simulink subsystem "TrajandControl"  (R2022a)
settings: Solver=VariableStepAuto  StartTime=0.0  StopTime=10.0  RelTol=1e-3
values from neighbouring files (symbols this model uses):
  kd_altitude = 0.475    [QuadcopterParameters.m]    (also in QuadcopterParameters1.m)
  kd_attitude = 20    [QuadcopterParameters.m]    (also in QuadcopterParameters1.m)
  KD_position = 0.85    [QuadcopterParameters.m]    (also in QuadcopterParameters1.m)
  ki_altitude = 0.275    [QuadcopterParameters.m]    (also in QuadcopterParameters1.m)
  ki_attitude = 0.01    [QuadcopterParameters.m]    (also in QuadcopterParameters1.m)
  KP_altitude = 0.8    [QuadcopterParameters.m]    (also in QuadcopterParameters1.m)
  kp_attitude = 1    [QuadcopterParameters.m]    (also in QuadcopterParameters1.m)
  KP_position = 0.1    [QuadcopterParameters.m]    (also in QuadcopterParameters1.m)
libraries: nesl_utility x6, slpidlib x4, sm_lib x1
settings Model: Creator=ADMIN  LastModifiedBy=ADMIN

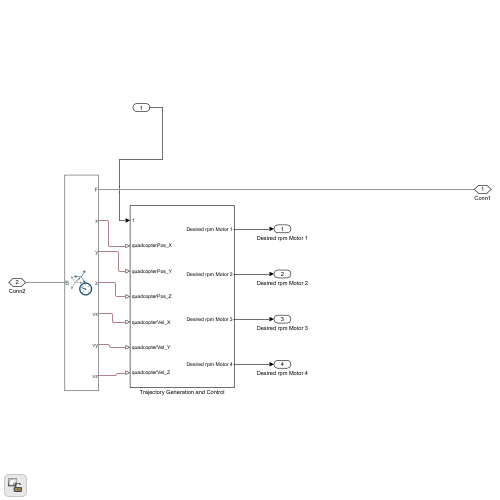
[thumbnail: Simulink's stored preview of the top-level diagram]
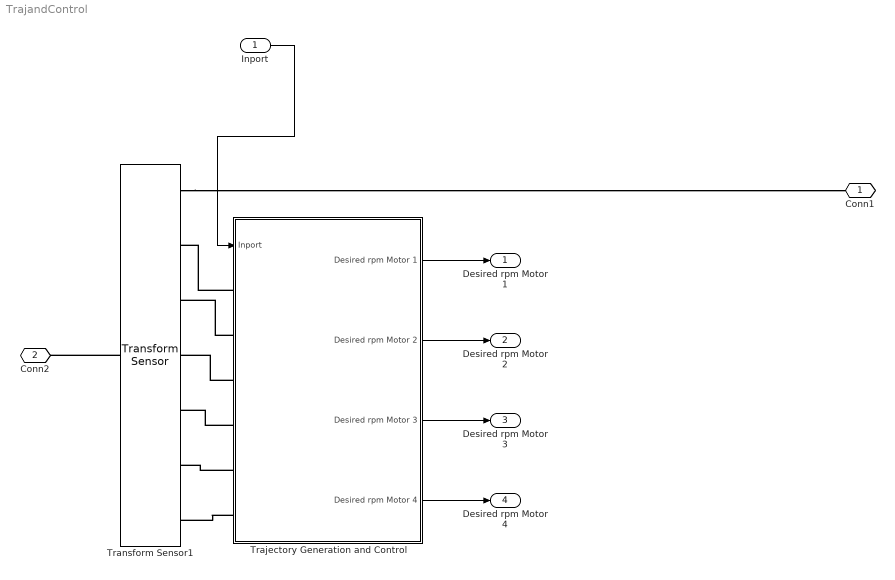
== system TrajandControl ==
  Inport : Inport
  Trajectory Generation and Control : Subsystem
  Transform Sensor1 : sm_lib/Frames and Transforms/Transform Sensor  MeasurementFrame=NonRotatingBase  SenseAngle=off  SenseAxis=off  SenseAngle1=off  SenseAngle2=off  SenseAngle3=off  SenseQ=off  SenseR=off  SenseOmegaX=off  SenseOmegaY=off  SenseOmegaZ=off  SenseOmega1=off  SenseOmega2=off  SenseOmega3=off  SenseQDot=off  SenseRDot=off  SenseAlphaX=off  SenseAlphaY=off  SenseAlphaZ=off  SenseAlpha1=off  SenseAlpha2=off  SenseAlpha3=off  SenseQDDot=off  SenseRDDot=off  SenseX=on  SenseY=on  SenseZ=on  SenseRad=off  SenseAzim=off  SenseDist=off  SenseInc=off  SenseXDot=on  SenseYDot=on  SenseZDot=on  SenseRadDot=off  SenseAzimDot=off  SenseDistDot=off  SenseIncDot=off  SenseXDDot=off  SenseYDDot=off  SenseZDDot=off  SenseRadDDot=off  SenseAzimDDot=off  SenseDistDDot=off  SenseIncDDot=off
  Conn1 : PMIOPort  Side=Right
  Conn2 : PMIOPort  Port=2  Side=Left
  Desired rpm Motor 1 : Outport
  Desired rpm Motor 2 : Outport  Port=2
  Desired rpm Motor 3 : Outport  Port=3
  Desired rpm Motor 4 : Outport  Port=4
  wires:
  Trajectory Generation and Control/2(Desired rpm Motor 2) -> Desired rpm Motor 2/1
  Inport/1 -> Trajectory Generation and Control/1(Inport)
  Trajectory Generation and Control/1(Desired rpm Motor 1) -> Desired rpm Motor 1/1
  Trajectory Generation and Control/3(Desired rpm Motor 3) -> Desired rpm Motor 3/1
  Trajectory Generation and Control/4(Desired rpm Motor 4) -> Desired rpm Motor 4/1
  connections:
  Trajectory Generation and Control/LConn1 -- Transform Sensor1/RConn2
  Trajectory Generation and Control/LConn5 -- Transform Sensor1/RConn6
  Trajectory Generation and Control/LConn3 -- Transform Sensor1/RConn4
  Trajectory Generation and Control/LConn2 -- Transform Sensor1/RConn3
  Trajectory Generation and Control/LConn6 -- Transform Sensor1/RConn7
  Trajectory Generation and Control/LConn4 -- Transform Sensor1/RConn5
  Transform Sensor1/LConn1 -- Conn2/RConn1
  Transform Sensor1/RConn1 -- Conn1/RConn1

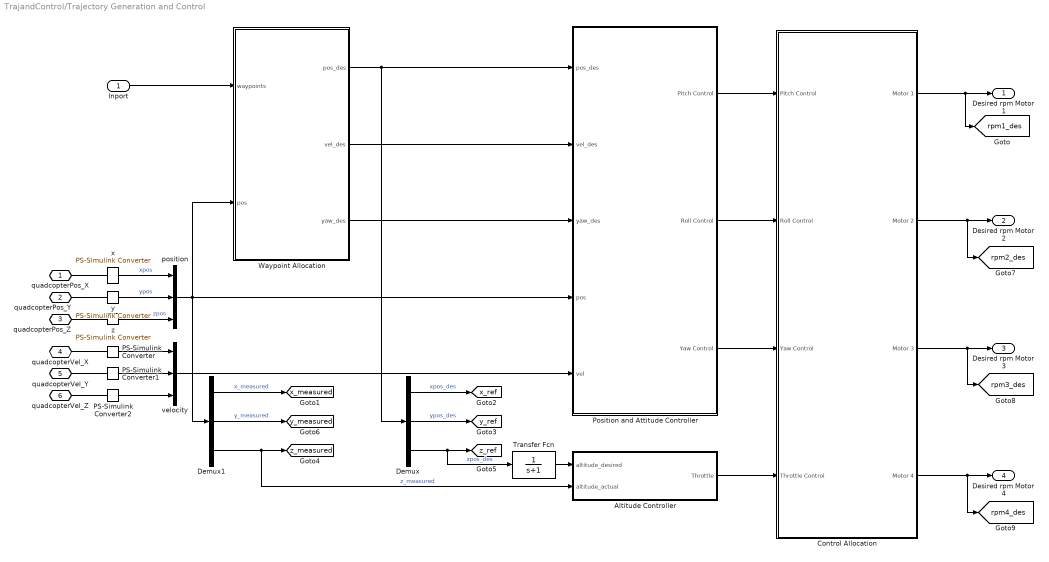
== system TrajandControl/Trajectory Generation and Control ==
  Inport : Inport
  Altitude Controller : Subsystem
  Control Allocation : Subsystem
  Demux : Demux  Outputs=3
  Demux1 : Demux  Outputs=3
  PS-Simulink Converter : nesl_utility/PS-Simulink Converter  PhysicalDomain=network_engine_domain  SubClassName=ps_output  LeftPortType=input  RightPortType=output  PseudoPeriodic=off  Frequencies=[]  VectorFormat=1-D array  Unit=inherit  AffineConversion=off
      settings: SourceProductBaseCode=SS,PW,VE
  PS-Simulink Converter1 : nesl_utility/PS-Simulink Converter  PhysicalDomain=network_engine_domain  SubClassName=ps_output  LeftPortType=input  RightPortType=output  PseudoPeriodic=off  Frequencies=[]  VectorFormat=1-D array  Unit=inherit  AffineConversion=off
      settings: SourceProductBaseCode=SS,PW,VE
  PS-Simulink Converter2 : nesl_utility/PS-Simulink Converter  PhysicalDomain=network_engine_domain  SubClassName=ps_output  LeftPortType=input  RightPortType=output  PseudoPeriodic=off  Frequencies=[]  VectorFormat=1-D array  Unit=inherit  AffineConversion=off
      settings: SourceProductBaseCode=SS,PW,VE
  Position and Attitude Controller : Subsystem
  Transfer Fcn : TransferFcn  Denominator=[1 1]
  Waypoint Allocation : MATLAB Function  TreatAsAtomicUnit=on
  position : Mux  Inputs=3
  velocity : Mux  Inputs=3
  x : nesl_utility/PS-Simulink Converter  PhysicalDomain=network_engine_domain  SubClassName=ps_output  LeftPortType=input  RightPortType=output  PseudoPeriodic=off  Frequencies=[]  VectorFormat=1-D array  Unit=1  AffineConversion=off
      settings: SourceProductBaseCode=SS,PW,VE
  y : nesl_utility/PS-Simulink Converter  PhysicalDomain=network_engine_domain  SubClassName=ps_output  LeftPortType=input  RightPortType=output  PseudoPeriodic=off  Frequencies=[]  VectorFormat=1-D array  Unit=1  AffineConversion=off
      settings: SourceProductBaseCode=SS,PW,VE
  z : nesl_utility/PS-Simulink Converter  PhysicalDomain=network_engine_domain  SubClassName=ps_output  LeftPortType=input  RightPortType=output  PseudoPeriodic=off  Frequencies=[]  VectorFormat=1-D array  Unit=1  AffineConversion=off
      settings: SourceProductBaseCode=SS,PW,VE
  quadcopterPos_X : PMIOPort  Side=Left
  quadcopterPos_Y : PMIOPort  Port=2  Side=Left
  quadcopterPos_Z : PMIOPort  Port=3  Side=Left
  quadcopterVel_X : PMIOPort  Port=4  Side=Left
  quadcopterVel_Y : PMIOPort  Port=5  Side=Left
  quadcopterVel_Z : PMIOPort  Port=6  Side=Left
  Desired rpm Motor 1 : Outport
  Desired rpm Motor 2 : Outport  Port=2
  Desired rpm Motor 3 : Outport  Port=3
  Desired rpm Motor 4 : Outport  Port=4
  tag scope: rpm1_des=global, rpm2_des=global, rpm3_des=global, rpm4_des=global, x_measured=global, x_ref=global, y_measured=global, y_ref=global, z_measured=global, z_ref=global
  wires:
  Control Allocation/4(Motor 4) -> Desired rpm Motor 4/1, [rpm4_des]
  Control Allocation/3(Motor 3) -> Desired rpm Motor 3/1, [rpm3_des]
  Control Allocation/1(Motor 1) -> [rpm1_des], Desired rpm Motor 1/1
  Transfer Fcn/1 -> Altitude Controller/1(altitude_desired)
  Inport/1 -> Waypoint Allocation/1(waypoints)
  Altitude Controller/1(Throttle) -> Control Allocation/4(Throttle Control)
  Position and Attitude Controller/3(Yaw Control) -> Control Allocation/3(Yaw Control)
  Position and Attitude Controller/1(Pitch Control) -> Control Allocation/1(Pitch Control)
  Position and Attitude Controller/2(Roll Control) -> Control Allocation/2(Roll Control)
  Waypoint Allocation/1(pos_des) -> Demux/1, Position and Attitude Controller/1(pos_des)
  Waypoint Allocation/2(vel_des) -> Position and Attitude Controller/2(vel_des)
  Waypoint Allocation/3(yaw_des) -> Position and Attitude Controller/3(yaw_des)
  Control Allocation/2(Motor 2) -> Desired rpm Motor 2/1, [rpm2_des]
  velocity/1 -> Position and Attitude Controller/5(vel)
  Demux1/2 -> [y_measured]  "y_measured"
  Demux1/3 -> Altitude Controller/2(altitude_actual), [z_measured]  "z_measured"
  Demux1/1 -> [x_measured]  "x_measured"
  y/1 -> position/2  "ypos"
  Demux/3 -> [z_ref], Transfer Fcn/1  "zpos_des"
  Demux/1 -> [x_ref]  "xpos_des"
  Demux/2 -> [y_ref]  "ypos_des"
  position/1 -> Position and Attitude Controller/4(pos), Demux1/1, Waypoint Allocation/2(pos)
  x/1 -> position/1  "xpos"
  PS-Simulink Converter2/1 -> velocity/3
  PS-Simulink Converter/1 -> velocity/1
  PS-Simulink Converter1/1 -> velocity/2
  z/1 -> position/3  "zpos"
  connections:
  quadcopterVel_Z/RConn1 -- PS-Simulink Converter2/LConn1
  PS-Simulink Converter1/LConn1 -- quadcopterVel_Y/RConn1
  z/LConn1 -- quadcopterPos_Z/RConn1
  PS-Simulink Converter/LConn1 -- quadcopterVel_X/RConn1
  x/LConn1 -- quadcopterPos_X/RConn1
  y/LConn1 -- quadcopterPos_Y/RConn1

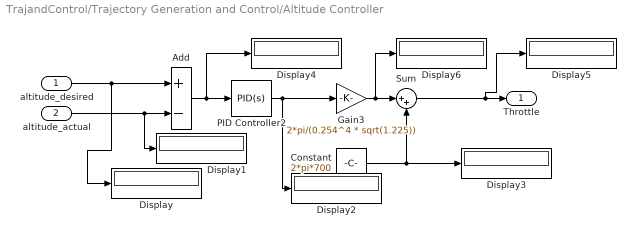
== system TrajandControl/Trajectory Generation and Control/Altitude Controller ==
  altitude_desired : Inport
  altitude_actual : Inport  Port=2
  Add : Sum  Inputs=+-
  Constant : Constant  Value=2*pi*700
  Display{,1..6} (7 alike) : Display
  Gain3 : Gain  Gain=2*pi/(0.254^4 * sqrt(1.225))
  PID Controller2 : slpidlib/PID Controller  Controller=PID  Form=Parallel  TimeDomain=Continuous-time  UseExternalTs=off  SampleTime=-1  IntegratorMethod=Forward Euler  FilterMethod=Forward Euler  ControllerParametersSource=internal  P=KP_altitude  I=ki_altitude  UseKiTs=off  D=kd_altitude  N=1000  UseFilter=on  TunerSelectOption=Transfer Function Based (PID Tuner App)  InitialConditionSource=internal  InitialConditionForIntegrator=0  InitialConditionForFilter=0  DifferentiatorICPrevScaledInput=0  ExternalReset=none  TrackingMode=off  Kt=1  LimitOutput=on  SatLimitsSource=internal  UpperSaturationLimit=50  LowerSaturationLimit=0  LinearizeAsGain=on  AntiWindupMode=none  Kb=1  POutMin=[]  POutMax=[]  IOutMin=[]  IOutMax=[]  DOutMin=[]  DOutMax=[]  NOutMin=[]  NOutMax=[]  SumOutMin=[]  SumOutMax=[]  SaturationOutMin=[]  SaturationOutMax=[]  PParamMin=[]  PParamMax=[]  IParamMin=[]  IParamMax=[]  DParamMin=[]  DParamMax=[]  NParamMin=[]  NParamMax=[]  KbParamMin=[]  KbParamMax=[]  KtParamMin=[]  KtParamMax=[]  KbOutMin=[]  KbOutMax=[]  KtOutMin=[]  KtOutMax=[]  IntegratorOutMin=[]  IntegratorOutMax=[]  FilterOutMin=[]  FilterOutMax=[]  SumI1OutMin=[]  SumI1OutMax=[]  SumI2OutMin=[]  SumI2OutMax=[]  SumI3OutMin=[]  SumI3OutMax=[]  SumI4OutMin=[]  SumI4OutMax=[]  SumDOutMin=[]  SumDOutMax=[]  DifferentiatorOutMin=[]  DifferentiatorOutMax=[]  FilterDiffOutCoefMin=[]  FilterDiffOutCoefMax=[]  ReciprocalOutMin=[]  ReciprocalOutMax=[]  SumDenOutMin=[]  SumDenOutMax=[]  SumNumOutMin=[]  SumNumOutMax=[]  DivideOutMin=[]  DivideOutMax=[]  UdiffTsProdOutMin=[]  UdiffTsProdOutMax=[]  NTsProdOutMin=[]  NTsProdOutMax=[]  UintegralTsProdOutMin=[]  UintegralTsProdOutMax=[]  UngainTsProdOutMin=[]  UngainTsProdOutMax=[]  IntegratorContinuousStateAttributes=''  IntegratorStateMustResolveToSignalObject=off  IntegratorRTWStateStorageClass=Auto  FilterContinuousStateAttributes=''  FilterStateMustResolveToSignalObject=off  FilterRTWStateStorageClass=Auto  ParallelPVariant=InternalParameters  IdealPVariant=Disabled  IVariant=InternalParameters  DVariant=InternalParameters  IntegratorVariant=Continuous  SatVariant=Enabled  AWVariant=Passthrough  PCopyVariant=Disabled  TRVariant=Disabled  FdbkBlocksVariant=Forward  IdealPFdbkVariant=Disabled  SatFdbkVariant=Disabled  DerivativeFilterVariant=ContFilter  NVariant=InternalParameters  NCopyVariant=Disabled  FilterICVariant=InternalICsFilter  IntegratorICVariant=InternalICs  ExternalResetVariant=Disabled  TRSumVariant=Passthrough  SumFdbkVariant=Disabled  SumVariant=Sum_PID  TsampFilterVariant=InternalTs  TsampNgainVariant=Passthrough  TsampIntegralVariant=Passthrough  ExternalSaturationOutDataTypeStr=Inherit: Same as second input  aMode=0
  Sum : Sum  Inputs=|++
  Throttle : Outport
  wires:
  Gain3/1 -> Sum/1, Display6/1
  altitude_desired/1 -> Add/1, Display/1
  Add/1 -> PID Controller2/1, Display4/1
  altitude_actual/1 -> Add/2, Display1/1
  PID Controller2/1 -> Gain3/1, Display2/1
  Constant/1 -> Sum/2, Display3/1
  Sum/1 -> Throttle/1, Display5/1

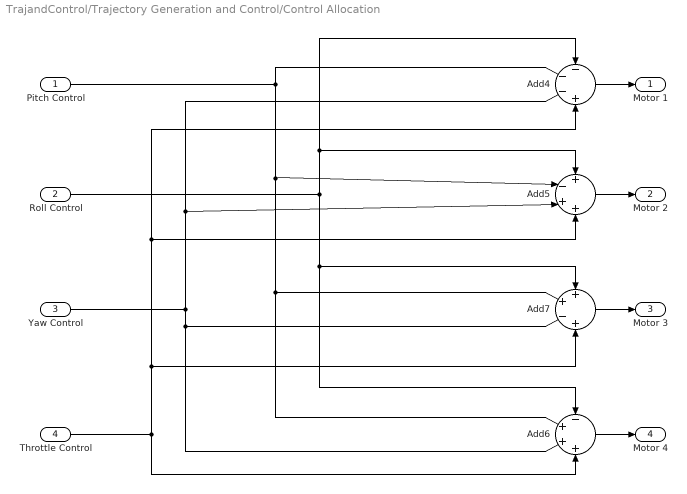
== system TrajandControl/Trajectory Generation and Control/Control Allocation ==
  Pitch Control : Inport
  Roll Control : Inport  Port=2
  Yaw Control : Inport  Port=3
  Throttle Control : Inport  Port=4
  Add4 : Sum  Inputs=---+
  Add5 : Sum  Inputs=+-++
  Add6 : Sum  Inputs=-+++
  Add7 : Sum  Inputs=++-+
  Motor 1 : Outport
  Motor 2 : Outport  Port=2
  Motor 3 : Outport  Port=3
  Motor 4 : Outport  Port=4
  wires:
  Throttle Control/1 -> Add5/4, Add4/4, Add7/4, Add6/4
  Yaw Control/1 -> Add5/3, Add4/3, Add7/3, Add6/3
  Pitch Control/1 -> Add5/2, Add7/2, Add6/2, Add4/2
  Roll Control/1 -> Add7/1, Add6/1, Add5/1, Add4/1
  Add5/1 -> Motor 2/1
  Add4/1 -> Motor 1/1
  Add6/1 -> Motor 4/1
  Add7/1 -> Motor 3/1

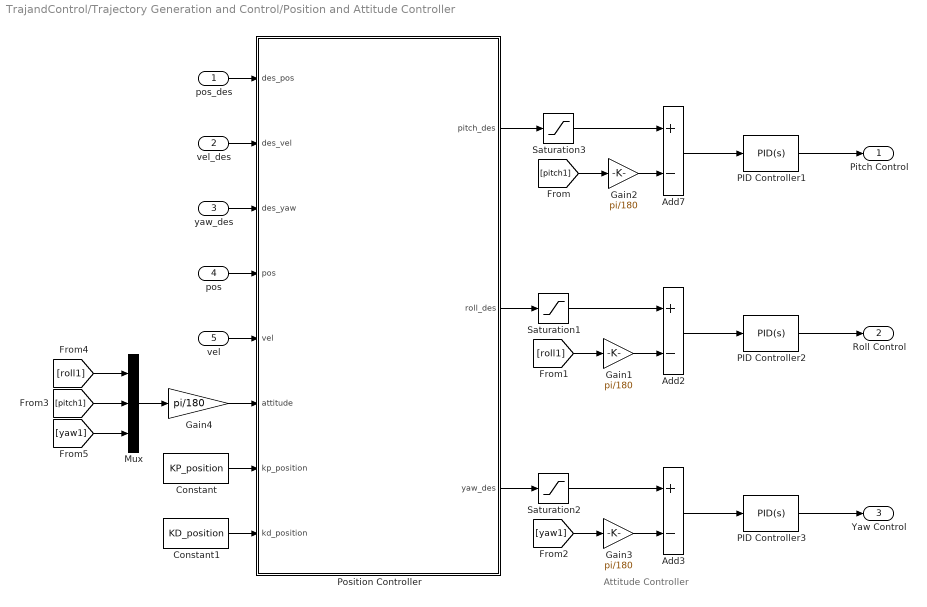
== system TrajandControl/Trajectory Generation and Control/Position and Attitude Controller ==
  note: Attitude Controller
  pos_des : Inport
  vel_des : Inport  Port=2
  yaw_des : Inport  Port=3
  pos : Inport  Port=4
  vel : Inport  Port=5
  Add2 : Sum  Inputs=+-
  Add3 : Sum  Inputs=+-
  Add7 : Sum  Inputs=+-
  Constant : Constant  Value=KP_position
  Constant1 : Constant  Value=KD_position
  Gain{1..4} (4 alike) : Gain  Gain=pi/180
  Mux : Mux  Inputs=3
  PID Controller1 : slpidlib/PID Controller  Controller=PID  Form=Parallel  TimeDomain=Continuous-time  UseExternalTs=off  SampleTime=-1  IntegratorMethod=Forward Euler  FilterMethod=Forward Euler  ControllerParametersSource=internal  P=kp_attitude  I=ki_attitude  UseKiTs=off  D=kd_attitude  N=100  UseFilter=on  TunerSelectOption=Transfer Function Based (PID Tuner App)  InitialConditionSource=internal  InitialConditionForIntegrator=0  InitialConditionForFilter=0  DifferentiatorICPrevScaledInput=0  ExternalReset=none  TrackingMode=off  Kt=1  LimitOutput=on  SatLimitsSource=internal  UpperSaturationLimit=20  LowerSaturationLimit=-20  LinearizeAsGain=on  AntiWindupMode=clamping  Kb=1  POutMin=[]  POutMax=[]  IOutMin=[]  IOutMax=[]  DOutMin=[]  DOutMax=[]  NOutMin=[]  NOutMax=[]  SumOutMin=[]  SumOutMax=[]  SaturationOutMin=[]  SaturationOutMax=[]  PParamMin=[]  PParamMax=[]  IParamMin=[]  IParamMax=[]  DParamMin=[]  DParamMax=[]  NParamMin=[]  NParamMax=[]  KbParamMin=[]  KbParamMax=[]  KtParamMin=[]  KtParamMax=[]  KbOutMin=[]  KbOutMax=[]  KtOutMin=[]  KtOutMax=[]  IntegratorOutMin=[]  IntegratorOutMax=[]  FilterOutMin=[]  FilterOutMax=[]  SumI1OutMin=[]  SumI1OutMax=[]  SumI2OutMin=[]  SumI2OutMax=[]  SumI3OutMin=[]  SumI3OutMax=[]  SumI4OutMin=[]  SumI4OutMax=[]  SumDOutMin=[]  SumDOutMax=[]  DifferentiatorOutMin=[]  DifferentiatorOutMax=[]  FilterDiffOutCoefMin=[]  FilterDiffOutCoefMax=[]  ReciprocalOutMin=[]  ReciprocalOutMax=[]  SumDenOutMin=[]  SumDenOutMax=[]  SumNumOutMin=[]  SumNumOutMax=[]  DivideOutMin=[]  DivideOutMax=[]  UdiffTsProdOutMin=[]  UdiffTsProdOutMax=[]  NTsProdOutMin=[]  NTsProdOutMax=[]  UintegralTsProdOutMin=[]  UintegralTsProdOutMax=[]  UngainTsProdOutMin=[]  UngainTsProdOutMax=[]  IntegratorContinuousStateAttributes=''  IntegratorStateMustResolveToSignalObject=off  IntegratorRTWStateStorageClass=Auto  FilterContinuousStateAttributes=''  FilterStateMustResolveToSignalObject=off  FilterRTWStateStorageClass=Auto  ParallelPVariant=InternalParameters  IdealPVariant=Disabled  IVariant=InternalParameters  DVariant=InternalParameters  IntegratorVariant=Continuous  SatVariant=Enabled  AWVariant=ContClampingParallel  PCopyVariant=Disabled  TRVariant=Disabled  FdbkBlocksVariant=Forward  IdealPFdbkVariant=Disabled  SatFdbkVariant=Disabled  DerivativeFilterVariant=ContFilter  NVariant=InternalParameters  NCopyVariant=Disabled  FilterICVariant=InternalICsFilter  IntegratorICVariant=InternalICs  ExternalResetVariant=Disabled  TRSumVariant=Passthrough  SumFdbkVariant=Disabled  SumVariant=Sum_PID  TsampFilterVariant=InternalTs  TsampNgainVariant=Passthrough  TsampIntegralVariant=Passthrough  ExternalSaturationOutDataTypeStr=Inherit: Same as second input  aMode=0
  PID Controller2 : slpidlib/PID Controller  Controller=PID  Form=Parallel  TimeDomain=Continuous-time  UseExternalTs=off  SampleTime=-1  IntegratorMethod=Forward Euler  FilterMethod=Forward Euler  ControllerParametersSource=internal  P=kp_attitude  I=ki_attitude  UseKiTs=off  D=kd_attitude  N=100  UseFilter=on  TunerSelectOption=Transfer Function Based (PID Tuner App)  InitialConditionSource=internal  InitialConditionForIntegrator=0  InitialConditionForFilter=0  DifferentiatorICPrevScaledInput=0  ExternalReset=none  TrackingMode=off  Kt=1  LimitOutput=on  SatLimitsSource=internal  UpperSaturationLimit=20  LowerSaturationLimit=-20  LinearizeAsGain=on  AntiWindupMode=clamping  Kb=1  POutMin=[]  POutMax=[]  IOutMin=[]  IOutMax=[]  DOutMin=[]  DOutMax=[]  NOutMin=[]  NOutMax=[]  SumOutMin=[]  SumOutMax=[]  SaturationOutMin=[]  SaturationOutMax=[]  PParamMin=[]  PParamMax=[]  IParamMin=[]  IParamMax=[]  DParamMin=[]  DParamMax=[]  NParamMin=[]  NParamMax=[]  KbParamMin=[]  KbParamMax=[]  KtParamMin=[]  KtParamMax=[]  KbOutMin=[]  KbOutMax=[]  KtOutMin=[]  KtOutMax=[]  IntegratorOutMin=[]  IntegratorOutMax=[]  FilterOutMin=[]  FilterOutMax=[]  SumI1OutMin=[]  SumI1OutMax=[]  SumI2OutMin=[]  SumI2OutMax=[]  SumI3OutMin=[]  SumI3OutMax=[]  SumI4OutMin=[]  SumI4OutMax=[]  SumDOutMin=[]  SumDOutMax=[]  DifferentiatorOutMin=[]  DifferentiatorOutMax=[]  FilterDiffOutCoefMin=[]  FilterDiffOutCoefMax=[]  ReciprocalOutMin=[]  ReciprocalOutMax=[]  SumDenOutMin=[]  SumDenOutMax=[]  SumNumOutMin=[]  SumNumOutMax=[]  DivideOutMin=[]  DivideOutMax=[]  UdiffTsProdOutMin=[]  UdiffTsProdOutMax=[]  NTsProdOutMin=[]  NTsProdOutMax=[]  UintegralTsProdOutMin=[]  UintegralTsProdOutMax=[]  UngainTsProdOutMin=[]  UngainTsProdOutMax=[]  IntegratorContinuousStateAttributes=''  IntegratorStateMustResolveToSignalObject=off  IntegratorRTWStateStorageClass=Auto  FilterContinuousStateAttributes=''  FilterStateMustResolveToSignalObject=off  FilterRTWStateStorageClass=Auto  ParallelPVariant=InternalParameters  IdealPVariant=Disabled  IVariant=InternalParameters  DVariant=InternalParameters  IntegratorVariant=Continuous  SatVariant=Enabled  AWVariant=ContClampingParallel  PCopyVariant=Disabled  TRVariant=Disabled  FdbkBlocksVariant=Forward  IdealPFdbkVariant=Disabled  SatFdbkVariant=Disabled  DerivativeFilterVariant=ContFilter  NVariant=InternalParameters  NCopyVariant=Disabled  FilterICVariant=InternalICsFilter  IntegratorICVariant=InternalICs  ExternalResetVariant=Disabled  TRSumVariant=Passthrough  SumFdbkVariant=Disabled  SumVariant=Sum_PID  TsampFilterVariant=InternalTs  TsampNgainVariant=Passthrough  TsampIntegralVariant=Passthrough  ExternalSaturationOutDataTypeStr=Inherit: Same as second input  aMode=0
  PID Controller3 : slpidlib/PID Controller  Controller=PID  Form=Parallel  TimeDomain=Continuous-time  UseExternalTs=off  SampleTime=-1  IntegratorMethod=Forward Euler  FilterMethod=Forward Euler  ControllerParametersSource=internal  P=kp_attitude  I=ki_attitude  UseKiTs=off  D=kd_attitude  N=100  UseFilter=on  TunerSelectOption=Transfer Function Based (PID Tuner App)  InitialConditionSource=internal  InitialConditionForIntegrator=0  InitialConditionForFilter=0  DifferentiatorICPrevScaledInput=0  ExternalReset=none  TrackingMode=off  Kt=1  LimitOutput=on  SatLimitsSource=internal  UpperSaturationLimit=50  LowerSaturationLimit=-50  LinearizeAsGain=on  AntiWindupMode=none  Kb=1  POutMin=[]  POutMax=[]  IOutMin=[]  IOutMax=[]  DOutMin=[]  DOutMax=[]  NOutMin=[]  NOutMax=[]  SumOutMin=[]  SumOutMax=[]  SaturationOutMin=[]  SaturationOutMax=[]  PParamMin=[]  PParamMax=[]  IParamMin=[]  IParamMax=[]  DParamMin=[]  DParamMax=[]  NParamMin=[]  NParamMax=[]  KbParamMin=[]  KbParamMax=[]  KtParamMin=[]  KtParamMax=[]  KbOutMin=[]  KbOutMax=[]  KtOutMin=[]  KtOutMax=[]  IntegratorOutMin=[]  IntegratorOutMax=[]  FilterOutMin=[]  FilterOutMax=[]  SumI1OutMin=[]  SumI1OutMax=[]  SumI2OutMin=[]  SumI2OutMax=[]  SumI3OutMin=[]  SumI3OutMax=[]  SumI4OutMin=[]  SumI4OutMax=[]  SumDOutMin=[]  SumDOutMax=[]  DifferentiatorOutMin=[]  DifferentiatorOutMax=[]  FilterDiffOutCoefMin=[]  FilterDiffOutCoefMax=[]  ReciprocalOutMin=[]  ReciprocalOutMax=[]  SumDenOutMin=[]  SumDenOutMax=[]  SumNumOutMin=[]  SumNumOutMax=[]  DivideOutMin=[]  DivideOutMax=[]  UdiffTsProdOutMin=[]  UdiffTsProdOutMax=[]  NTsProdOutMin=[]  NTsProdOutMax=[]  UintegralTsProdOutMin=[]  UintegralTsProdOutMax=[]  UngainTsProdOutMin=[]  UngainTsProdOutMax=[]  IntegratorContinuousStateAttributes=''  IntegratorStateMustResolveToSignalObject=off  IntegratorRTWStateStorageClass=Auto  FilterContinuousStateAttributes=''  FilterStateMustResolveToSignalObject=off  FilterRTWStateStorageClass=Auto  ParallelPVariant=InternalParameters  IdealPVariant=Disabled  IVariant=InternalParameters  DVariant=InternalParameters  IntegratorVariant=Continuous  SatVariant=Enabled  AWVariant=Passthrough  PCopyVariant=Disabled  TRVariant=Disabled  FdbkBlocksVariant=Forward  IdealPFdbkVariant=Disabled  SatFdbkVariant=Disabled  DerivativeFilterVariant=ContFilter  NVariant=InternalParameters  NCopyVariant=Disabled  FilterICVariant=InternalICsFilter  IntegratorICVariant=InternalICs  ExternalResetVariant=Disabled  TRSumVariant=Passthrough  SumFdbkVariant=Disabled  SumVariant=Sum_PID  TsampFilterVariant=InternalTs  TsampNgainVariant=Passthrough  TsampIntegralVariant=Passthrough  ExternalSaturationOutDataTypeStr=Inherit: Same as second input  aMode=0
  Position Controller : MATLAB Function  TreatAsAtomicUnit=on
  Saturation1 : Saturate  UpperLimit=pi/3  LowerLimit=-pi/3
  Saturation2 : Saturate  UpperLimit=pi/3  LowerLimit=-pi/3
  Saturation3 : Saturate  UpperLimit=pi/3  LowerLimit=-pi/3
  Pitch Control : Outport
  Roll Control : Outport  Port=2
  Yaw Control : Outport  Port=3
  wires:
  PID Controller2/1 -> Roll Control/1
  PID Controller1/1 -> Pitch Control/1
  PID Controller3/1 -> Yaw Control/1
  Constant1/1 -> Position Controller/8(kd_position)
  Constant/1 -> Position Controller/7(kp_position)
  Add3/1 -> PID Controller3/1
  Add2/1 -> PID Controller2/1
  Add7/1 -> PID Controller1/1
  Gain2/1 -> Add7/2
  Gain3/1 -> Add3/2
  Gain1/1 -> Add2/2
  Gain4/1 -> Position Controller/6(attitude)
  [yaw1] -> Mux/3
  [pitch1] -> Mux/2
  [roll1] -> Mux/1
  Mux/1 -> Gain4/1
  Position Controller/1(pitch_des) -> Saturation3/1
  Saturation3/1 -> Add7/1
  Saturation1/1 -> Add2/1
  vel_des/1 -> Position Controller/2(des_vel)
  [pitch1] -> Gain2/1
  [roll1] -> Gain1/1
  [yaw1] -> Gain3/1
  vel/1 -> Position Controller/5(vel)
  yaw_des/1 -> Position Controller/3(des_yaw)
  Position Controller/3(yaw_des) -> Saturation2/1
  Saturation2/1 -> Add3/1
  Position Controller/2(roll_des) -> Saturation1/1
  pos_des/1 -> Position Controller/1(des_pos)
  pos/1 -> Position Controller/4(pos)

== matlab function TrajandControl/Trajectory Generation and Control/Position and Attitude Controller/Position Controller ==
  data: des_pos input; des_vel input; des_yaw input; pos input; vel input; pitch_des output; roll_des output; yaw_des output; attitude input; kp_position input; kd_position input
function [pitch_des,roll_des,yaw_des] = position_controller(des_pos,des_vel,des_yaw,pos,vel,attitude, kp_position, kd_position)
% This MATLAB function computes the desired roll, pitch and yaw angles to
% control the position of the quadcopter.

% Euler Angles
phi = attitude(1);
theta = attitude(2);
psi = attitude(3);

%% Obtain the desired state

% Direction Cosine Matrix
DCM = [cos(theta)*cos(psi)                                    cos(theta)*sin(psi)                          -sin(theta);
    -cos(phi)*sin(psi)+sin(phi)*sin(theta)*cos(psi) cos(phi)*cos(psi)+sin(phi)*sin(theta)*sin(psi) sin(phi)*cos(theta);
    sin(phi)*sin(psi)+cos(phi)*sin(theta)*cos(psi) -sin(phi)*cos(psi)+cos(phi)*sin(theta)*sin(psi) cos(phi)*cos(theta)];

% Desired Velocity
v_des = DCM*((des_vel - vel) + kp_position*(des_pos - pos));

% Desired Roll, Pitch and Yaw
pitch_des = (1/(9.81))*(kd_position*v_des(1)); 
roll_des = (-1/(9.81))*(kd_position*v_des(2)); 
yaw_des = des_yaw;
end

== matlab function TrajandControl/Trajectory Generation and Control/Waypoint Allocation ==
  settings: updateMethod=DISCRETE
  data: pos_des output; vel_des output; yaw_des output; waypoints input; pos input
% function [pos_des, vel_des, yaw_des, counter, dist] = trajectory_generator(t, homePose, timespot, waypoints, pos)
function [pos_des, vel_des, yaw_des] = trajectory_generator(waypoints, pos)
coder.extrinsic('containers.Map');
% This MATLAB function is used to calculate the desired trajectory for the
% quadcopter.

persistent distance2waypoint waypointCounter;
persistent state keySet valueSet M;



% Calculate the desired trajectory from the home position to the first waypoint
if isempty(waypointCounter)
   waypointCounter = 1;
   keySet = {'Hover','Follow'};
   valueSet = [0 1];
   M = containers.Map(keySet,valueSet);
   state = M('Follow');
%    counter = 0;
   % Distance to the First Waypoint
   distance2waypoint = sqrt(sum((pos-waypoints(:,waypointCounter)).^2));
end


%% If the quadcopter is within the proximity of the Waypoint, compute the trajectory from the current waypoint to the next waypoint
while (distance2waypoint <= 5) && state
   % Update the waypointCounter
   waypointCounter = waypointCounter + 1;
   if waypointCounter < length(waypoints)
      distance2waypoint = sqrt(sum((pos-waypoints(:,waypointCounter)).^2));
   else
      state = M('Hover');
   end
end

%% If the quadcopter has reached the target, then hover at the target location
if waypointCounter > length(waypoints)
   pos_des = waypoints(:,end);
   vel_des = (pos_des - pos)/5;
else
   pos_des = waypoints(:,waypointCounter);
   vel_des = (pos_des - pos)/5; %0.1*ones(3,1)+[0;0;0];
   for i = 1:3
      if(abs(vel_des(i)) > 2)
         vel_des(i) = 2*sign(vel_des(i));
      end
   end
   distance2waypoint = sqrt(sum((pos-waypoints(:,waypointCounter)).^2));
end

%% Desired Heading Angle
yaw_des = 0;
% t
% counter = waypointCounter
% dist = distance2waypoint
end
